simulink model "cohenCoonPI"  (R2023b)
settings: Solver=VariableStepAuto  StartTime=0.0  StopTime=10.0  RelTol=1e-3
settings Model: Creator=usuario  LastModifiedBy=usuario
settings DataIOCC: ReturnWorkspaceOutputs=off

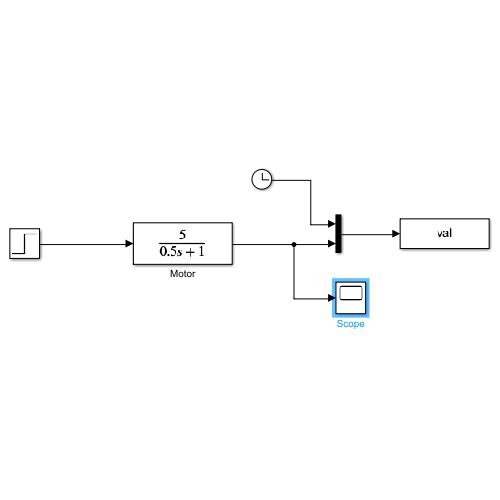
[thumbnail: Simulink's stored preview of the top-level diagram]
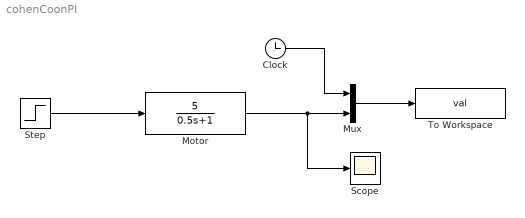
== system cohenCoonPI ==
  Clock : Clock
  Motor : TransferFcn  Numerator=[5]  Denominator=[0.5 1]
  Mux : Mux  Inputs=2
  Scope : Scope
  Step : Step  After=12  SampleTime=0
  To Workspace : ToWorkspace  VariableName=val  SampleTime=0.01
  wires:
  Step/1 -> Motor/1
  Mux/1 -> To Workspace/1
  Motor/1 -> Scope/1, Mux/2
  Clock/1 -> Mux/1
